simulink model "sampleModel7"  (R2021a)
settings: Solver=VariableStepAuto  StartTime=0.0  StopTime=10.0  RelTol=1e-3
undefined symbols (not defined in the file): DiscIntNeverNeededParam, magnitude, Newton, Raphson
libraries: simulink x210, pid_lib x47, simulink_need_slupdate x2
(part 7 of 8)

== system sampleModel7/cfblk364/cfblk6/cfblk16/cfblk5 ==
  cfblk1 : Inport
  cfblk15 : Inport  Port=2
  cfblk16 : Inport  Port=3
  cfblk10 : Sum  Inputs=|++
  cfblk11 : Sqrt  SaturateOnIntegerOverflow=on
  cfblk12 : Sin  TimeSource=Use external signal  SampleTime=0
  cfblk13 : Reshape
  cfblk14 : Sqrt  Operator=rSqrt  AlgorithmType=Newton-Raphson  SaturateOnIntegerOverflow=on
  cfblk17 : Delay
  cfblk3 : simulink/Discrete/Difference  ICPrevInput=0.0  OutMin=[]  OutMax=[]  OutDataTypeStr=Inherit: Inherit via back propagation  OutDataType=fixdt(1, 16)  OutScaling=2^-10  DoSatur=off
  cfblk4 : simulink/Discrete/Tapped Delay  vinit=0.0  samptime=-1  NumDelays=1  DelayOrder=Oldest  includeCurrent=off
  cfblk5 : DiscreteZeroPole  Poles=[0 0.5]  Gain=1  SampleTime=-1
  cfblk6 : Sqrt  Operator=rSqrt  AlgorithmType=Newton-Raphson  SaturateOnIntegerOverflow=on
  cfblk7 : Sum  Inputs=+-
  cfblk8 : DotProduct  InputSameDT=on  OutDataTypeStr=Inherit: Inherit via internal rule
  cfblk9 : MinMax  Function=max
  cfblk2 : Outport
  wires:
  cfblk13/1 -> cfblk10/1
  cfblk5/1 -> cfblk10/2
  cfblk11/1 -> cfblk7/1
  cfblk7/1 -> cfblk5/1
  cfblk16/1 -> cfblk6/1
  cfblk3/1 -> cfblk13/1, cfblk8/2
  cfblk12/1 -> cfblk2/1
  cfblk6/1 -> cfblk3/1
  cfblk9/1 -> cfblk12/1
  cfblk14/1 -> cfblk9/1
  cfblk15/1 -> cfblk14/1
  cfblk4/1 -> cfblk8/1
  cfblk1/1 -> cfblk4/1
  cfblk8/1 -> cfblk11/1
  cfblk10/1 -> cfblk17/1
  cfblk17/1 -> cfblk7/2

== system sampleModel7/cfblk364/cfblk6/cfblk16/cfblk6 ==
  cfblk1 : Inport
  cfblk7 : Inport  Port=2
  cfblk10 : Delay
  cfblk11 : Delay
  cfblk12 : Delay
  cfblk3 : DiscreteFir
  cfblk4 : Delay  DelayLengthSource=Input port
      settings: InputPortMap=u0,p1
  cfblk5 : Constant  Value=[426363474.539316]  SampleTime=1
  cfblk6 : If  IfExpression=u1 >= 0  SampleTime=1
  cfblk8 : Subsystem  TreatAsAtomicUnit=on
  cfblk9 : Subsystem  TreatAsAtomicUnit=on
  cfblk2 : Outport
  wires:
  cfblk1/1 -> cfblk9/2(cfblk12)
  cfblk7/1 -> cfblk9/3(cfblk13)
  cfblk5/1 -> cfblk6/1, cfblk8/2(cfblk14)
  cfblk9/1(cfblk2) -> cfblk4/2
  cfblk4/1 -> cfblk2/1, cfblk10/1
  cfblk9/2(cfblk14) -> cfblk8/1(cfblk1), cfblk8/3(cfblk15)
  cfblk8/2(cfblk17) -> cfblk3/1
  cfblk6/1 -> cfblk8/Action
  cfblk6/2 -> cfblk9/Action
  cfblk10/1 -> cfblk8/4(cfblk16)
  cfblk8/1(cfblk2) -> cfblk11/1
  cfblk11/1 -> cfblk9/1(cfblk1)
  cfblk3/1 -> cfblk12/1
  cfblk12/1 -> cfblk4/1

== system sampleModel7/cfblk382/cfblk17/cfblk13/cfblk6 ==
  cfblk1 : Inport
  cfblk7 : Inport  Port=2
  cfblk8 : Inport  Port=3
  cfblk3 : UnitDelay  SampleTime=-1  HasFrameUpgradeWarning=on
  cfblk4 : pid_lib/PID Controller  Controller=PID  Form=Parallel  TimeDomain=Discrete-time  UseExternalTs=off  SampleTime=-1  IntegratorMethod=Forward Euler  FilterMethod=Forward Euler  ControllerParametersSource=internal  P=1  I=1  D=0  UseFilter=on  N=100  TunerSelectOption=Transfer Function Based (PID Tuner App)  InitialConditionSource=internal  InitialConditionForIntegrator=0  InitialConditionForFilter=0  DifferentiatorICPrevScaledInput=0  ExternalReset=none  TrackingMode=off  Kt=1  LimitOutput=off  SatLimitsSource=internal  UpperSaturationLimit=inf  LowerSaturationLimit=-inf  LinearizeAsGain=off  AntiWindupMode=none  Kb=1  POutMin=[]  POutMax=[]  IOutMin=[]  IOutMax=[]  DOutMin=[]  DOutMax=[]  NOutMin=[]  NOutMax=[]  SumOutMin=[]  SumOutMax=[]  SaturationOutMin=[]  SaturationOutMax=[]  PParamMin=[]  PParamMax=[]  IParamMin=[]  IParamMax=[]  DParamMin=[]  DParamMax=[]  NParamMin=[]  NParamMax=[]  KbParamMin=[]  KbParamMax=[]  KtParamMin=[]  KtParamMax=[]  KbOutMin=[]  KbOutMax=[]  KtOutMin=[]  KtOutMax=[]  IntegratorOutMin=[]  IntegratorOutMax=[]  FilterOutMin=[]  FilterOutMax=[]  SumI1OutMin=[]  SumI1OutMax=[]  SumI2OutMin=[]  SumI2OutMax=[]  SumI3OutMin=[]  SumI3OutMax=[]  SumI4OutMin=[]  SumI4OutMax=[]  SumDOutMin=[]  SumDOutMax=[]  DifferentiatorOutMin=[]  DifferentiatorOutMax=[]  FilterDiffOutCoefMin=[]  FilterDiffOutCoefMax=[]  ReciprocalOutMin=[]  ReciprocalOutMax=[]  SumDenOutMin=[]  SumDenOutMax=[]  SumNumOutMin=[]  SumNumOutMax=[]  DivideOutMin=[]  DivideOutMax=[]  UdiffTsProdOutMin=[]  UdiffTsProdOutMax=[]  NTsProdOutMin=[]  NTsProdOutMax=[]  UintegralTsProdOutMin=[]  UintegralTsProdOutMax=[]  UngainTsProdOutMin=[]  UngainTsProdOutMax=[]  IntegratorContinuousStateAttributes=''  IntegratorStateMustResolveToSignalObject=off  IntegratorRTWStateStorageClass=Auto  FilterContinuousStateAttributes=''  FilterStateMustResolveToSignalObject=off  FilterRTWStateStorageClass=Auto  ParallelPVariant=InternalParameters  IdealPVariant=Disabled  IVariant=InternalParameters  DVariant=InternalParameters  IntegratorVariant=Discrete  SatVariant=Disabled  AWVariant=Passthrough  PCopyVariant=Disabled  TRVariant=Disabled  FdbkBlocksVariant=Forward  IdealPFdbkVariant=Disabled  SatFdbkVariant=Disabled  DerivativeFilterVariant=ForwardEulerFilter  NVariant=InternalParameters  NCopyVariant=Disabled  FilterICVariant=InternalICsFilter  IntegratorICVariant=InternalICs  ExternalResetVariant=Disabled  TRSumVariant=Passthrough  SumFdbkVariant=Disabled  SumVariant=Sum_PID  TsampFilterVariant=InternalTs  TsampNgainVariant=Passthrough  TsampIntegralVariant=Passthrough  ExternalSaturationOutDataTypeStr=Inherit: Same as second input
  cfblk5 : Sum  Inputs=+
  cfblk6 : Subsystem
  cfblk2 : Outport
  wires:
  cfblk1/1 -> cfblk6/1(cfblk1)
  cfblk4/1 -> cfblk5/1
  cfblk5/1 -> cfblk2/1
  cfblk7/1 -> cfblk6/2(cfblk9)
  cfblk6/1(cfblk2) -> cfblk3/1
  cfblk3/1 -> cfblk4/1

== system sampleModel7/cfblk384/cfblk14/cfblk8/cfblk11 ==
  cfblk1 : Inport
  cfblk8 : Inport  Port=2
  cfblk9 : Inport  Port=3
  cfblk10 : Inport  Port=4
  cfblk12 : Delay
  cfblk3 : Delay
  cfblk4 : DiscreteStateSpace  SampleTime=-1
  cfblk5 : DotProduct  InputSameDT=on  OutDataTypeStr=Inherit: Inherit via internal rule
  cfblk6 : Assignment  DiagnosticForDimensions=Warning  IndexOptions=Index vector (dialog)  Indices=1  OutputSizes=1
  cfblk7 : Constant  Value=[822552432.782879]  SampleTime=1
  cfblk2 : Outport
  cfblk11 : Outport  Port=2
  wires:
  cfblk7/1 -> cfblk2/1
  cfblk10/1 -> cfblk4/1
  cfblk1/1 -> cfblk11/1
  cfblk6/1 -> cfblk5/1
  cfblk4/1 -> cfblk3/1
  cfblk3/1 -> cfblk6/2
  cfblk9/1 -> cfblk5/2
  cfblk5/1 -> cfblk12/1
  cfblk12/1 -> cfblk6/1

== system sampleModel7/cfblk396/cfblk6/cfblk13/cfblk13 ==
  cfblk1 : Inport
  cfblk10 : Inport  Port=2
  cfblk11 : Inport  Port=3
  cfblk12 : Inport  Port=4
  cfblk3 : simulink/Discrete/Difference  ICPrevInput=0.0  OutMin=[]  OutMax=[]  OutDataTypeStr=Inherit: Inherit via back propagation  OutDataType=fixdt(1, 16)  OutScaling=2^-10  DoSatur=off
  cfblk4 : DiscreteFilter
  cfblk5 : Math  Operator=10^u  SaturateOnIntegerOverflow=on
  cfblk6 : Sum  Inputs=--
  cfblk7 : MinMax  Function=max  Inputs=3
  cfblk8 : Constant  Value=[446745629.042101]  SampleTime=1
  cfblk9 : Subsystem
  cfblk2 : Outport
  wires:
  cfblk4/1 -> cfblk9/1(cfblk1)
  cfblk10/1 -> cfblk6/1, cfblk7/3
  cfblk7/1 -> cfblk3/1
  cfblk8/1 -> cfblk7/1
  cfblk9/1(cfblk2) -> cfblk6/2
  cfblk12/1 -> cfblk5/1
  cfblk5/1 -> cfblk4/1
  cfblk3/1 -> cfblk9/2(cfblk8)
  cfblk6/1 -> cfblk2/1
  cfblk1/1 -> cfblk9/3(cfblk9)
  cfblk11/1 -> cfblk7/2

== system sampleModel7/cfblk399/cfblk15/cfblk6/cfblk8 ==
  cfblk1 : Inport
  cfblk10 : Inport  Port=2
  cfblk11 : Inport  Port=3
  cfblk12 : Inport  Port=4
  cfblk13 : Inport  Port=5
  cfblk14 : Inport  Port=6
  cfblk15 : DataTypeConversion
  cfblk3 : simulink/Discrete/Transfer Fcn First Order  PoleZ=0.95  ICPrevOutput=0.0  DoSatur=off
  cfblk4 : pid_lib/PID Controller  Controller=PID  Form=Parallel  TimeDomain=Discrete-time  UseExternalTs=off  SampleTime=-1  IntegratorMethod=Forward Euler  FilterMethod=Forward Euler  ControllerParametersSource=internal  P=1  I=1  D=0  UseFilter=on  N=100  TunerSelectOption=Transfer Function Based (PID Tuner App)  InitialConditionSource=internal  InitialConditionForIntegrator=0  InitialConditionForFilter=0  DifferentiatorICPrevScaledInput=0  ExternalReset=none  TrackingMode=off  Kt=1  LimitOutput=off  SatLimitsSource=internal  UpperSaturationLimit=inf  LowerSaturationLimit=-inf  LinearizeAsGain=off  AntiWindupMode=none  Kb=1  POutMin=[]  POutMax=[]  IOutMin=[]  IOutMax=[]  DOutMin=[]  DOutMax=[]  NOutMin=[]  NOutMax=[]  SumOutMin=[]  SumOutMax=[]  SaturationOutMin=[]  SaturationOutMax=[]  PParamMin=[]  PParamMax=[]  IParamMin=[]  IParamMax=[]  DParamMin=[]  DParamMax=[]  NParamMin=[]  NParamMax=[]  KbParamMin=[]  KbParamMax=[]  KtParamMin=[]  KtParamMax=[]  KbOutMin=[]  KbOutMax=[]  KtOutMin=[]  KtOutMax=[]  IntegratorOutMin=[]  IntegratorOutMax=[]  FilterOutMin=[]  FilterOutMax=[]  SumI1OutMin=[]  SumI1OutMax=[]  SumI2OutMin=[]  SumI2OutMax=[]  SumI3OutMin=[]  SumI3OutMax=[]  SumI4OutMin=[]  SumI4OutMax=[]  SumDOutMin=[]  SumDOutMax=[]  DifferentiatorOutMin=[]  DifferentiatorOutMax=[]  FilterDiffOutCoefMin=[]  FilterDiffOutCoefMax=[]  ReciprocalOutMin=[]  ReciprocalOutMax=[]  SumDenOutMin=[]  SumDenOutMax=[]  SumNumOutMin=[]  SumNumOutMax=[]  DivideOutMin=[]  DivideOutMax=[]  UdiffTsProdOutMin=[]  UdiffTsProdOutMax=[]  NTsProdOutMin=[]  NTsProdOutMax=[]  UintegralTsProdOutMin=[]  UintegralTsProdOutMax=[]  UngainTsProdOutMin=[]  UngainTsProdOutMax=[]  IntegratorContinuousStateAttributes=''  IntegratorStateMustResolveToSignalObject=off  IntegratorRTWStateStorageClass=Auto  FilterContinuousStateAttributes=''  FilterStateMustResolveToSignalObject=off  FilterRTWStateStorageClass=Auto  ParallelPVariant=InternalParameters  IdealPVariant=Disabled  IVariant=InternalParameters  DVariant=InternalParameters  IntegratorVariant=Discrete  SatVariant=Disabled  AWVariant=Passthrough  PCopyVariant=Disabled  TRVariant=Disabled  FdbkBlocksVariant=Forward  IdealPFdbkVariant=Disabled  SatFdbkVariant=Disabled  DerivativeFilterVariant=ForwardEulerFilter  NVariant=InternalParameters  NCopyVariant=Disabled  FilterICVariant=InternalICsFilter  IntegratorICVariant=InternalICs  ExternalResetVariant=Disabled  TRSumVariant=Passthrough  SumFdbkVariant=Disabled  SumVariant=Sum_PID  TsampFilterVariant=InternalTs  TsampNgainVariant=Passthrough  TsampIntegralVariant=Passthrough  ExternalSaturationOutDataTypeStr=Inherit: Same as second input
  cfblk5 : Product  Inputs=*
  cfblk6 : UnaryMinus
  cfblk7 : Constant  Value=[-757788657.864586]  SampleTime=1
  cfblk8 : Constant  Value=[-711690762.176715]  SampleTime=1
  cfblk9 : Constant  Value=[91822789.155668]  SampleTime=1
  cfblk2 : Outport
  wires:
  cfblk9/1 -> cfblk3/1
  cfblk7/1 -> cfblk6/1
  cfblk14/1 -> cfblk5/1
  cfblk3/1 -> cfblk2/1
  cfblk1/1 -> cfblk15/1
  cfblk15/1 -> cfblk4/1

== system sampleModel7/cfblk403/cfblk9/cfblk8/cfblk12 ==
  cfblk1 : Inport
  cfblk11 : Inport  Port=2
  cfblk12 : Inport  Port=3
  cfblk13 : Inport  Port=4
  cfblk14 : Inport  Port=5
  cfblk10 : Constant  Value=[-534013201.984926]  SampleTime=1
  cfblk3 : pid_lib/PID Controller  Controller=PID  Form=Parallel  TimeDomain=Discrete-time  UseExternalTs=off  SampleTime=-1  IntegratorMethod=Forward Euler  FilterMethod=Forward Euler  ControllerParametersSource=internal  P=1  I=1  D=0  UseFilter=on  N=100  TunerSelectOption=Transfer Function Based (PID Tuner App)  InitialConditionSource=internal  InitialConditionForIntegrator=0  InitialConditionForFilter=0  DifferentiatorICPrevScaledInput=0  ExternalReset=none  TrackingMode=off  Kt=1  LimitOutput=off  SatLimitsSource=internal  UpperSaturationLimit=inf  LowerSaturationLimit=-inf  LinearizeAsGain=off  AntiWindupMode=none  Kb=1  POutMin=[]  POutMax=[]  IOutMin=[]  IOutMax=[]  DOutMin=[]  DOutMax=[]  NOutMin=[]  NOutMax=[]  SumOutMin=[]  SumOutMax=[]  SaturationOutMin=[]  SaturationOutMax=[]  PParamMin=[]  PParamMax=[]  IParamMin=[]  IParamMax=[]  DParamMin=[]  DParamMax=[]  NParamMin=[]  NParamMax=[]  KbParamMin=[]  KbParamMax=[]  KtParamMin=[]  KtParamMax=[]  KbOutMin=[]  KbOutMax=[]  KtOutMin=[]  KtOutMax=[]  IntegratorOutMin=[]  IntegratorOutMax=[]  FilterOutMin=[]  FilterOutMax=[]  SumI1OutMin=[]  SumI1OutMax=[]  SumI2OutMin=[]  SumI2OutMax=[]  SumI3OutMin=[]  SumI3OutMax=[]  SumI4OutMin=[]  SumI4OutMax=[]  SumDOutMin=[]  SumDOutMax=[]  DifferentiatorOutMin=[]  DifferentiatorOutMax=[]  FilterDiffOutCoefMin=[]  FilterDiffOutCoefMax=[]  ReciprocalOutMin=[]  ReciprocalOutMax=[]  SumDenOutMin=[]  SumDenOutMax=[]  SumNumOutMin=[]  SumNumOutMax=[]  DivideOutMin=[]  DivideOutMax=[]  UdiffTsProdOutMin=[]  UdiffTsProdOutMax=[]  NTsProdOutMin=[]  NTsProdOutMax=[]  UintegralTsProdOutMin=[]  UintegralTsProdOutMax=[]  UngainTsProdOutMin=[]  UngainTsProdOutMax=[]  IntegratorContinuousStateAttributes=''  IntegratorStateMustResolveToSignalObject=off  IntegratorRTWStateStorageClass=Auto  FilterContinuousStateAttributes=''  FilterStateMustResolveToSignalObject=off  FilterRTWStateStorageClass=Auto  ParallelPVariant=InternalParameters  IdealPVariant=Disabled  IVariant=InternalParameters  DVariant=InternalParameters  IntegratorVariant=Discrete  SatVariant=Disabled  AWVariant=Passthrough  PCopyVariant=Disabled  TRVariant=Disabled  FdbkBlocksVariant=Forward  IdealPFdbkVariant=Disabled  SatFdbkVariant=Disabled  DerivativeFilterVariant=ForwardEulerFilter  NVariant=InternalParameters  NCopyVariant=Disabled  FilterICVariant=InternalICsFilter  IntegratorICVariant=InternalICs  ExternalResetVariant=Disabled  TRSumVariant=Passthrough  SumFdbkVariant=Disabled  SumVariant=Sum_PID  TsampFilterVariant=InternalTs  TsampNgainVariant=Passthrough  TsampIntegralVariant=Passthrough  ExternalSaturationOutDataTypeStr=Inherit: Same as second input
  cfblk4 : Bias  Bias=[542628662.857885]
  cfblk5 : Bias  Bias=[-760541575.504912]
  cfblk6 : Polyval  Coefs=[ +2.081618890e-019, -1.441693666e-014, +4.719686976e-010, -8.536869453e-006, +1.621573104e-001, -8.087801117e+001 ]
  cfblk7 : Sqrt  SaturateOnIntegerOverflow=on
  cfblk8 : UnaryMinus
  cfblk9 : MinMax  Function=max  Inputs=2
  cfblk2 : Outport
  wires:
  cfblk8/1 -> cfblk9/1
  cfblk10/1 -> cfblk8/1
  cfblk1/1 -> cfblk4/1
  cfblk12/1 -> cfblk2/1
  cfblk11/1 -> cfblk7/1
  cfblk13/1 -> cfblk6/1
  cfblk4/1 -> cfblk9/2
  cfblk9/1 -> cfblk5/1
  cfblk14/1 -> cfblk3/1

== system sampleModel7/cfblk349/cfblk10/cfblk10/cfblk10/cfblk13 ==
  cfblk1 : Inport
  cfblk9 : Inport  Port=2
  cfblk10 : Delay  SampleTime=1
  cfblk3 : Delay  ShowEnablePort=on  SampleTime=1
      settings: InputPortMap=u0,e6
  cfblk4 : Signum
  cfblk5 : Product
  cfblk6 : ComplexToMagnitudeAngle
  cfblk7 : Product  Inputs=**
  cfblk8 : Constant  Value=[-509073102.910421]  SampleTime=1
  cfblk2 : Outport
  wires:
  cfblk7/1 -> cfblk6/1
  cfblk6/1 -> cfblk5/1
  cfblk5/1 -> cfblk3/1
  cfblk8/1 -> cfblk3/2
  cfblk4/1 -> cfblk5/2
  cfblk9/1 -> cfblk4/1
  cfblk1/1 -> cfblk7/2
  cfblk3/1 -> cfblk2/1
  cfblk6/2 -> cfblk10/1
  cfblk10/1 -> cfblk7/1

== system sampleModel7/cfblk349/cfblk10/cfblk10/cfblk10/cfblk14 ==
  cfblk1 : Inport
  cfblk3 : Sin  TimeSource=Use external signal  SampleTime=0
  cfblk4 : Signum
  cfblk5 : UnaryMinus
  cfblk6 : Constant  Value=[-85370784.622687]  SampleTime=1
  cfblk7 : Constant  Value=[764398997.464723]  SampleTime=1
  cfblk2 : Outport
  wires:
  cfblk7/1 -> cfblk5/1
  cfblk1/1 -> cfblk3/1
  cfblk6/1 -> cfblk4/1
  cfblk4/1 -> cfblk2/1

== system sampleModel7/cfblk349/cfblk10/cfblk9/cfblk6/cfblk7 ==
  cfblk1 : Inport
  cfblk10 : Inport  Port=2
  cfblk11 : Inport  Port=3
  cfblk12 : Inport  Port=4
  cfblk3 : pid_lib/PID Controller (2DOF)  Controller=PID  Form=Parallel  TimeDomain=Discrete-time  UseExternalTs=off  SampleTime=1  IntegratorMethod=Forward Euler  FilterMethod=Forward Euler  ControllerParametersSource=internal  P=1  I=1  D=0  UseFilter=on  N=100  b=1  c=1  TunerSelectOption=Transfer Function Based (PID Tuner App)  InitialConditionSource=internal  InitialConditionForIntegrator=0  InitialConditionForFilter=0  DifferentiatorICPrevScaledInput=0  ExternalReset=none  TrackingMode=off  Kt=1  LimitOutput=off  SatLimitsSource=internal  UpperSaturationLimit=inf  LowerSaturationLimit=-inf  LinearizeAsGain=off  AntiWindupMode=none  Kb=1  POutMin=[]  POutMax=[]  IOutMin=[]  IOutMax=[]  DOutMin=[]  DOutMax=[]  NOutMin=[]  NOutMax=[]  bOutMin=[]  bOutMax=[]  cOutMin=[]  cOutMax=[]  SumOutMin=[]  SumOutMax=[]  SaturationOutMin=[]  SaturationOutMax=[]  PParamMin=[]  PParamMax=[]  IParamMin=[]  IParamMax=[]  DParamMin=[]  DParamMax=[]  NParamMin=[]  NParamMax=[]  bParamMin=[]  bParamMax=[]  cParamMin=[]  cParamMax=[]  KbParamMin=[]  KbParamMax=[]  KtParamMin=[]  KtParamMax=[]  KbOutMin=[]  KbOutMax=[]  KtOutMin=[]  KtOutMax=[]  IntegratorOutMin=[]  IntegratorOutMax=[]  FilterOutMin=[]  FilterOutMax=[]  SumI1OutMin=[]  SumI1OutMax=[]  SumI2OutMin=[]  SumI2OutMax=[]  SumI3OutMin=[]  SumI3OutMax=[]  SumI4OutMin=[]  SumI4OutMax=[]  SumDOutMin=[]  SumDOutMax=[]  Sum1OutMin=[]  Sum1OutMax=[]  Sum2OutMin=[]  Sum2OutMax=[]  Sum3OutMin=[]  Sum3OutMax=[]  DifferentiatorOutMin=[]  DifferentiatorOutMax=[]  FilterDiffOutCoefMin=[]  FilterDiffOutCoefMax=[]  ReciprocalOutMin=[]  ReciprocalOutMax=[]  SumDenOutMin=[]  SumDenOutMax=[]  SumNumOutMin=[]  SumNumOutMax=[]  DivideOutMin=[]  DivideOutMax=[]  UdiffTsProdOutMin=[]  UdiffTsProdOutMax=[]  NTsProdOutMin=[]  NTsProdOutMax=[]  UintegralTsProdOutMin=[]  UintegralTsProdOutMax=[]  UngainTsProdOutMin=[]  UngainTsProdOutMax=[]  IntegratorContinuousStateAttributes=''  IntegratorStateMustResolveToSignalObject=off  IntegratorRTWStateStorageClass=Auto  FilterContinuousStateAttributes=''  FilterStateMustResolveToSignalObject=off  FilterRTWStateStorageClass=Auto  ParallelPVariant=InternalParameters  IdealPVariant=Disabled  IVariant=InternalParameters  DVariant=InternalParameters  bVariant=InternalParameters  cVariant=InternalParameters  IntegratorVariant=Discrete  SatVariant=Disabled  AWVariant=Passthrough  PCopyVariant=Disabled  TRVariant=Disabled  FdbkBlocksVariant=Forward  IdealPFdbkVariant=Disabled  SatFdbkVariant=Disabled  DerivativeFilterVariant=ForwardEulerFilter  NVariant=InternalParameters  NCopyVariant=Disabled  FilterICVariant=InternalICsFilter  IntegratorICVariant=InternalICs  ExternalResetVariant=Disabled  TRSumVariant=Passthrough  SumFdbkVariant=Disabled  SumVariant=Sum_PID  TsampFilterVariant=InternalTs  TsampNgainVariant=Passthrough  TsampIntegralVariant=Passthrough  ExternalSaturationOutDataTypeStr=Inherit: Same as second input
      settings: SourceProductBaseCode=SL
  cfblk4 : DiscreteStateSpace
  cfblk5 : Delay  SampleTime=1
  cfblk6 : DiscreteFilter  SampleTime=1
  cfblk7 : simulink/Discrete/Transfer Fcn First Order  PoleZ=0.95  ICPrevOutput=0.0  DoSatur=off
  cfblk8 : Sin  TimeSource=Use external signal  SampleTime=0
  cfblk9 : simulink/Math Operations/MinMax Running Resettable  Function=min  vinit=0.0
  cfblk2 : Outport
  wires:
  cfblk12/1 -> cfblk7/1
  cfblk6/1 -> cfblk8/1
  cfblk1/1 -> cfblk4/1
  cfblk7/1 -> cfblk9/1
  cfblk5/1 -> cfblk6/1
  cfblk10/1 -> cfblk9/2
  cfblk9/1 -> cfblk3/1
  cfblk8/1 -> cfblk2/1
  cfblk11/1 -> cfblk3/2
  cfblk3/1 -> cfblk5/1

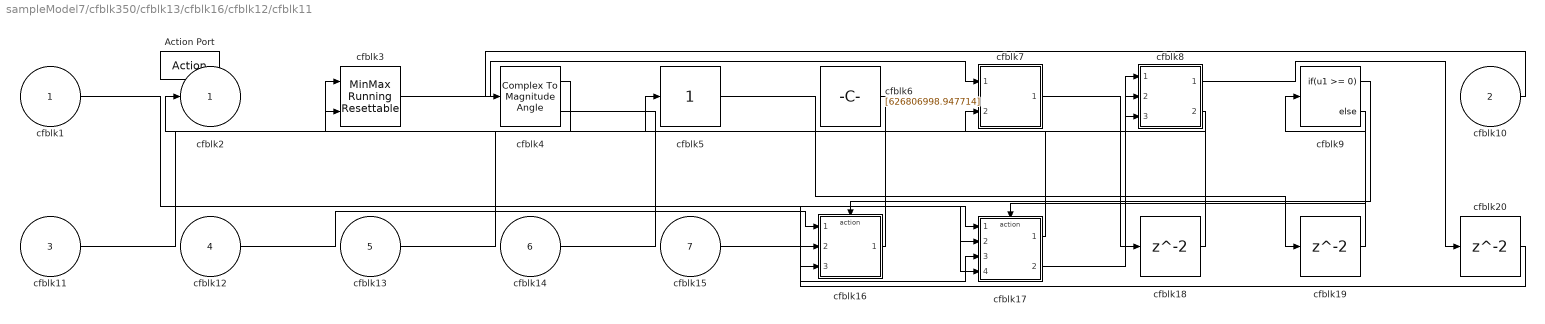
== system sampleModel7/cfblk350/cfblk13/cfblk16/cfblk12/cfblk11 ==
  cfblk1 : Inport
  cfblk10 : Inport  Port=2
  cfblk11 : Inport  Port=3
  cfblk12 : Inport  Port=4
  cfblk13 : Inport  Port=5
  cfblk14 : Inport  Port=6
  cfblk15 : Inport  Port=7
  Action Port : ActionPort  ActionPortLabel=if(u1 >= 0)
  cfblk16 : Subsystem  TreatAsAtomicUnit=on
  cfblk17 : Subsystem  TreatAsAtomicUnit=on
  cfblk18 : Delay
  cfblk19 : Delay
  cfblk20 : Delay
  cfblk3 : simulink/Math Operations/MinMax Running Resettable  Function=min  vinit=0.0
  cfblk4 : ComplexToMagnitudeAngle
  cfblk5 : simulink/Math Operations/Slider Gain  gain=1  low=0  high=2
  cfblk6 : Constant  Value=[626806998.947714]  SampleTime=1
  cfblk7 : Subsystem
  cfblk8 : Subsystem
  cfblk9 : If  IfExpression=u1 >= 0  SampleTime=1
  cfblk2 : Outport
  wires:
  cfblk17/1(cfblk2) -> cfblk5/1
  cfblk3/1 -> cfblk7/1(cfblk1)
  cfblk12/1 -> cfblk16/1(cfblk1)
  cfblk4/1 -> cfblk2/1
  cfblk10/1 -> cfblk4/1
  cfblk8/2(cfblk9) -> cfblk7/2(cfblk9)
  cfblk6/1 -> cfblk16/3(cfblk8)
  cfblk1/1 -> cfblk17/1(cfblk1)
  cfblk11/1 -> cfblk8/1(cfblk1)
  cfblk13/1 -> cfblk8/2(cfblk7)
  cfblk14/1 -> cfblk17/2(cfblk12)
  cfblk17/2(cfblk15) -> cfblk8/3(cfblk8)
  cfblk16/1(cfblk2) -> cfblk3/1
  cfblk15/1 -> cfblk17/3(cfblk13)
  cfblk4/2 -> cfblk17/4(cfblk14)
  cfblk9/1 -> cfblk16/Action
  cfblk9/2 -> cfblk17/Action
  cfblk7/1(cfblk2) -> cfblk18/1
  cfblk18/1 -> cfblk3/2
  cfblk5/1 -> cfblk19/1
  cfblk19/1 -> cfblk9/1
  cfblk8/1(cfblk2) -> cfblk20/1
  cfblk20/1 -> cfblk16/2(cfblk7)

== system sampleModel7/cfblk350/cfblk13/cfblk16/cfblk12/cfblk12 ==
  cfblk1 : Inport
  cfblk6 : Inport  Port=2
  cfblk7 : Inport  Port=3
  cfblk8 : Inport  Port=4
  cfblk9 : Inport  Port=5
  cfblk10 : Inport  Port=6
  Action Port : ActionPort  ActionPortLabel=else
  cfblk3 : UnaryMinus
  cfblk4 : Sum  Inputs=|++
  cfblk5 : Polyval  Coefs=[ +2.081618890e-019, -1.441693666e-014, +4.719686976e-010, -8.536869453e-006, +1.621573104e-001, -8.087801117e+001 ]
  cfblk2 : Outport
  wires:
  cfblk8/1 -> cfblk2/1
  cfblk3/1 -> cfblk4/1
  cfblk10/1 -> cfblk5/1
  cfblk9/1 -> cfblk4/2
  cfblk1/1 -> cfblk3/1

== system sampleModel7/cfblk350/cfblk13/cfblk17/cfblk6/cfblk18 ==
  cfblk1 : Inport
  cfblk11 : Inport  Port=2
  cfblk12 : Inport  Port=3
  cfblk13 : Inport  Port=4
  cfblk14 : Inport  Port=5
  cfblk15 : Inport  Port=6
  Action Port : ActionPort  ActionPortLabel=if(u1 >= 0)
  cfblk10 : Subsystem
  cfblk16 : Delay
  cfblk17 : Delay
  cfblk3 : DiscreteZeroPole  Poles=[0 0.5]  Gain=1  SampleTime=-1
  cfblk4 : Delay  DelayLengthSource=Input port
      settings: InputPortMap=u0,p1
  cfblk5 : Assignment  DiagnosticForDimensions=Warning  IndexOptions=Index vector (dialog)  Indices=1  OutputSizes=1
  cfblk6 : Sum  Inputs=+
  cfblk7 : Assignment  DiagnosticForDimensions=Warning  IndexOptions=Index vector (dialog)  Indices=1  OutputSizes=1
  cfblk8 : simulink/Math Operations/Slider Gain  gain=1  low=0  high=2
  cfblk9 : Constant  Value=[-20660821.855437]  SampleTime=1
  cfblk2 : Outport
  wires:
  cfblk8/1 -> cfblk2/1
  cfblk15/1 -> cfblk5/1
  cfblk4/1 -> cfblk7/2
  cfblk5/1 -> cfblk8/1
  cfblk13/1 -> cfblk5/2
  cfblk11/1 -> cfblk3/1
  cfblk3/1 -> cfblk10/1(cfblk1)
  cfblk1/1 -> cfblk10/2(cfblk8)
  cfblk7/1 -> cfblk6/1, cfblk16/1
  cfblk10/1(cfblk2) -> cfblk4/1
  cfblk14/1 -> cfblk10/4(cfblk10)
  cfblk9/1 -> cfblk4/2
  cfblk12/1 -> cfblk10/5(cfblk11)
  cfblk16/1 -> cfblk10/3(cfblk9)
  cfblk6/1 -> cfblk17/1
  cfblk17/1 -> cfblk7/1

== system sampleModel7/cfblk350/cfblk13/cfblk17/cfblk6/cfblk19 ==
  cfblk1 : Inport
  cfblk11 : Inport  Port=2
  cfblk12 : Inport  Port=3
  cfblk13 : Inport  Port=4
  cfblk14 : Inport  Port=5
  cfblk15 : Inport  Port=6
  Action Port : ActionPort  ActionPortLabel=else
  cfblk10 : Subsystem
  cfblk16 : Delay
  cfblk17 : Delay
  cfblk18 : Delay
  cfblk3 : DiscreteFilter
  cfblk4 : Delay  DelayLengthSource=Input port
      settings: InputPortMap=u0,p1
  cfblk5 : ComplexToRealImag
  cfblk6 : Signum
  cfblk7 : Bias  Bias=[41415960.158917]
  cfblk8 : Bias  Bias=[195329552.760084]
  cfblk9 : Subsystem
  cfblk2 : Outport
  wires:
  cfblk13/1 -> cfblk2/1
  cfblk15/1 -> cfblk4/1
  cfblk10/1(cfblk2) -> cfblk4/2
  cfblk1/1 -> cfblk6/1
  cfblk5/1 -> cfblk8/1
  cfblk11/1 -> cfblk10/1(cfblk1)
  cfblk5/2 -> cfblk3/1
  cfblk10/2(cfblk9) -> cfblk9/2(cfblk6)
  cfblk7/1 -> cfblk9/3(cfblk7)
  cfblk14/1 -> cfblk7/1
  cfblk9/1(cfblk2) -> cfblk5/1
  cfblk12/1 -> cfblk9/4(cfblk8)
  cfblk6/1 -> cfblk10/3(cfblk7)
  cfblk4/1 -> cfblk16/1
  cfblk16/1 -> cfblk10/2(cfblk6)
  cfblk8/1 -> cfblk17/1
  cfblk17/1 -> cfblk9/1(cfblk1)
  cfblk3/1 -> cfblk18/1
  cfblk18/1 -> cfblk10/4(cfblk8)

== system sampleModel7/cfblk353/cfblk8/cfblk11/cfblk7/cfblk6 ==
  cfblk1 : Inport
  cfblk11 : Inport  Port=2
  cfblk12 : Inport  Port=3
  cfblk13 : Inport  Port=4
  cfblk10 : If  IfExpression=u1 >= 0  SampleTime=1
  cfblk14 : Subsystem  TreatAsAtomicUnit=on
  cfblk15 : Subsystem  TreatAsAtomicUnit=on
  cfblk{5,16..18} (4 alike) : Delay  SampleTime=1
  cfblk3 : UnitDelay  HasFrameUpgradeWarning=on
  cfblk4 : simulink/Discrete/Difference  ICPrevInput=0.0  OutMin=[]  OutMax=[]  OutDataTypeStr=Inherit: Inherit via back propagation  OutDataType=fixdt(1, 16)  OutScaling=2^-10  DoSatur=off
  cfblk6 : Sum  Inputs=+
  cfblk7 : PermuteDimensions
  cfblk8 : MinMax  Inputs=3
  cfblk9 : DotProduct  InputSameDT=on  OutDataTypeStr=Inherit: Inherit via internal rule
  cfblk2 : Outport
  wires:
  cfblk14/1(cfblk2) -> cfblk6/1, cfblk18/1
  cfblk13/1 -> cfblk15/1(cfblk1)
  cfblk4/1 -> cfblk3/1, cfblk14/2(cfblk4)
  cfblk7/1 -> cfblk14/1(cfblk1)
  cfblk11/1 -> cfblk15/2(cfblk6), cfblk8/3, cfblk14/3(cfblk5), cfblk15/7(cfblk11)
  cfblk5/1 -> cfblk7/1
  cfblk3/1 -> cfblk15/3(cfblk7), cfblk2/1, cfblk14/5(cfblk7)
  cfblk12/1 -> cfblk5/1, cfblk15/4(cfblk8), cfblk15/5(cfblk9), cfblk14/4(cfblk6)
  cfblk1/1 -> cfblk9/1, cfblk15/6(cfblk10), cfblk15/8(cfblk12)
  cfblk9/1 -> cfblk8/2, cfblk15/9(cfblk13)
  cfblk8/1 -> cfblk4/1
  cfblk10/1 -> cfblk14/Action
  cfblk10/2 -> cfblk15/Action
  cfblk15/1(cfblk2) -> cfblk16/1
  cfblk16/1 -> cfblk9/2
  cfblk6/1 -> cfblk17/1
  cfblk17/1 -> cfblk8/1
  cfblk18/1 -> cfblk10/1

== system sampleModel7/cfblk354/cfblk18/cfblk11/cfblk8/cfblk14 ==
  cfblk1 : Inport
  cfblk3 : UnitDelay  SampleTime=-1  HasFrameUpgradeWarning=on
  cfblk4 : pid_lib/PID Controller  Controller=PID  Form=Parallel  TimeDomain=Discrete-time  UseExternalTs=off  SampleTime=-1  IntegratorMethod=Forward Euler  FilterMethod=Forward Euler  ControllerParametersSource=internal  P=1  I=1  D=0  UseFilter=on  N=100  TunerSelectOption=Transfer Function Based (PID Tuner App)  InitialConditionSource=internal  InitialConditionForIntegrator=0  InitialConditionForFilter=0  DifferentiatorICPrevScaledInput=0  ExternalReset=none  TrackingMode=off  Kt=1  LimitOutput=off  SatLimitsSource=internal  UpperSaturationLimit=inf  LowerSaturationLimit=-inf  LinearizeAsGain=off  AntiWindupMode=none  Kb=1  POutMin=[]  POutMax=[]  IOutMin=[]  IOutMax=[]  DOutMin=[]  DOutMax=[]  NOutMin=[]  NOutMax=[]  SumOutMin=[]  SumOutMax=[]  SaturationOutMin=[]  SaturationOutMax=[]  PParamMin=[]  PParamMax=[]  IParamMin=[]  IParamMax=[]  DParamMin=[]  DParamMax=[]  NParamMin=[]  NParamMax=[]  KbParamMin=[]  KbParamMax=[]  KtParamMin=[]  KtParamMax=[]  KbOutMin=[]  KbOutMax=[]  KtOutMin=[]  KtOutMax=[]  IntegratorOutMin=[]  IntegratorOutMax=[]  FilterOutMin=[]  FilterOutMax=[]  SumI1OutMin=[]  SumI1OutMax=[]  SumI2OutMin=[]  SumI2OutMax=[]  SumI3OutMin=[]  SumI3OutMax=[]  SumI4OutMin=[]  SumI4OutMax=[]  SumDOutMin=[]  SumDOutMax=[]  DifferentiatorOutMin=[]  DifferentiatorOutMax=[]  FilterDiffOutCoefMin=[]  FilterDiffOutCoefMax=[]  ReciprocalOutMin=[]  ReciprocalOutMax=[]  SumDenOutMin=[]  SumDenOutMax=[]  SumNumOutMin=[]  SumNumOutMax=[]  DivideOutMin=[]  DivideOutMax=[]  UdiffTsProdOutMin=[]  UdiffTsProdOutMax=[]  NTsProdOutMin=[]  NTsProdOutMax=[]  UintegralTsProdOutMin=[]  UintegralTsProdOutMax=[]  UngainTsProdOutMin=[]  UngainTsProdOutMax=[]  IntegratorContinuousStateAttributes=''  IntegratorStateMustResolveToSignalObject=off  IntegratorRTWStateStorageClass=Auto  FilterContinuousStateAttributes=''  FilterStateMustResolveToSignalObject=off  FilterRTWStateStorageClass=Auto  ParallelPVariant=InternalParameters  IdealPVariant=Disabled  IVariant=InternalParameters  DVariant=InternalParameters  IntegratorVariant=Discrete  SatVariant=Disabled  AWVariant=Passthrough  PCopyVariant=Disabled  TRVariant=Disabled  FdbkBlocksVariant=Forward  IdealPFdbkVariant=Disabled  SatFdbkVariant=Disabled  DerivativeFilterVariant=ForwardEulerFilter  NVariant=InternalParameters  NCopyVariant=Disabled  FilterICVariant=InternalICsFilter  IntegratorICVariant=InternalICs  ExternalResetVariant=Disabled  TRSumVariant=Passthrough  SumFdbkVariant=Disabled  SumVariant=Sum_PID  TsampFilterVariant=InternalTs  TsampNgainVariant=Passthrough  TsampIntegralVariant=Passthrough  ExternalSaturationOutDataTypeStr=Inherit: Same as second input
  cfblk5 : DiscreteStateSpace  SampleTime=-1
  cfblk6 : ComplexToRealImag
  cfblk7 : UnaryMinus
  cfblk8 : Delay
  cfblk2 : Outport
  wires:
  cfblk6/1 -> cfblk5/1
  cfblk7/1 -> cfblk6/1
  cfblk1/1 -> cfblk4/1
  cfblk3/1 -> cfblk7/1
  cfblk5/1 -> cfblk2/1
  cfblk6/2 -> cfblk8/1
  cfblk8/1 -> cfblk3/1

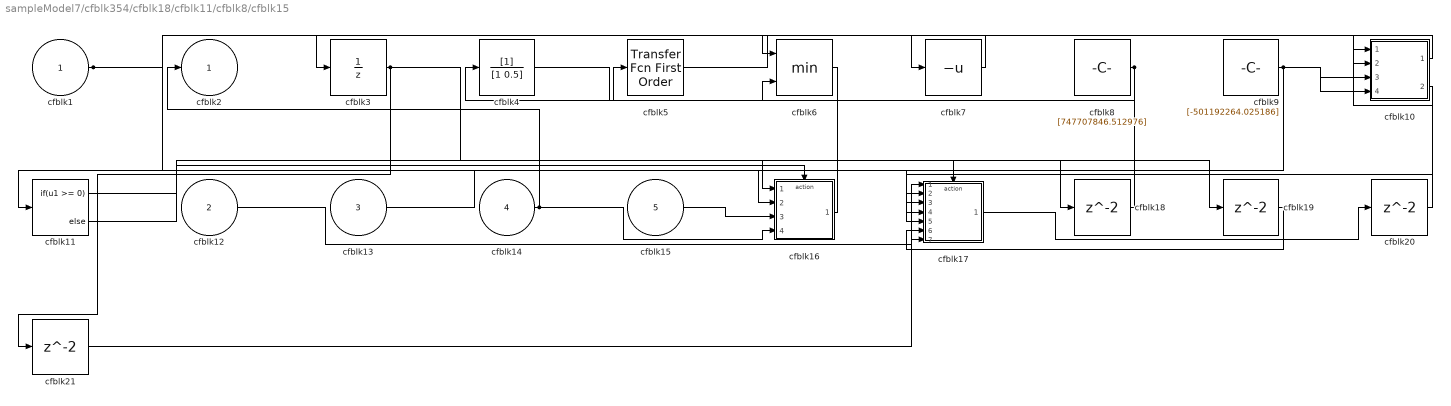
== system sampleModel7/cfblk354/cfblk18/cfblk11/cfblk8/cfblk15 ==
  cfblk1 : Inport
  cfblk12 : Inport  Port=2
  cfblk13 : Inport  Port=3
  cfblk14 : Inport  Port=4
  cfblk15 : Inport  Port=5
  cfblk10 : Subsystem
  cfblk11 : If  IfExpression=u1 >= 0  SampleTime=1
  cfblk16 : Subsystem  TreatAsAtomicUnit=on
  cfblk17 : Subsystem  TreatAsAtomicUnit=on
  cfblk{18..21} (4 alike) : Delay
  cfblk3 : UnitDelay  SampleTime=-1  HasFrameUpgradeWarning=on
  cfblk4 : DiscreteFilter
  cfblk5 : simulink/Discrete/Transfer Fcn First Order  PoleZ=0.95  ICPrevOutput=0.0  DoSatur=off
  cfblk6 : MinMax  Inputs=2
  cfblk7 : UnaryMinus
  cfblk8 : Constant  Value=[747707846.512976]  SampleTime=1
  cfblk9 : Constant  Value=[-501192264.025186]  SampleTime=1
  cfblk2 : Outport
  wires:
  cfblk7/1 -> cfblk3/1
  cfblk8/1 -> cfblk4/1, cfblk17/5(cfblk15)
  cfblk14/1 -> cfblk2/1, cfblk16/4(cfblk8)
  cfblk12/1 -> cfblk17/1(cfblk1)
  cfblk5/1 -> cfblk7/1
  cfblk3/1 -> cfblk18/1, cfblk19/1, cfblk21/1
  cfblk10/1(cfblk2) -> cfblk6/1
  cfblk6/1 -> cfblk11/1
  cfblk16/1(cfblk2) -> cfblk5/1
  cfblk4/1 -> cfblk6/2
  cfblk9/1 -> cfblk16/2(cfblk6), cfblk10/3(cfblk9), cfblk10/4(cfblk10)
  cfblk13/1 -> cfblk17/2(cfblk12)
  cfblk1/1 -> cfblk10/2(cfblk8), cfblk17/4(cfblk14)
  cfblk15/1 -> cfblk16/3(cfblk7)
  cfblk10/2(cfblk11) -> cfblk17/3(cfblk13)
  cfblk11/1 -> cfblk16/Action
  cfblk11/2 -> cfblk17/Action
  cfblk18/1 -> cfblk16/1(cfblk1)
  cfblk19/1 -> cfblk17/6(cfblk16)
  cfblk17/1(cfblk2) -> cfblk20/1
  cfblk20/1 -> cfblk10/1(cfblk1)
  cfblk21/1 -> cfblk17/7(cfblk17)

== system sampleModel7/cfblk364/cfblk6/cfblk16/cfblk4/cfblk15 ==
  cfblk1 : Inport
  cfblk10 : Inport  Port=2
  cfblk11 : Inport  Port=3
  Action Port : ActionPort  ActionPortLabel=if(u1 >= 0)
  cfblk12 : Delay
  cfblk3 : simulink/Discrete/Transfer Fcn First Order  PoleZ=0.95  ICPrevOutput=0.0  DoSatur=off
  cfblk4 : Sum  Inputs=-+
  cfblk5 : Product
  cfblk6 : Reshape
  cfblk7 : Reshape
  cfblk8 : Product  Inputs=*
  cfblk9 : Subsystem
  cfblk2 : Outport
  wires:
  cfblk6/1 -> cfblk2/1, cfblk9/3(cfblk9), cfblk9/4(cfblk10)
  cfblk11/1 -> cfblk5/1
  cfblk7/1 -> cfblk5/2
  cfblk1/1 -> cfblk4/2
  cfblk3/1 -> cfblk8/1
  cfblk10/1 -> cfblk3/1, cfblk9/2(cfblk8), cfblk9/5(cfblk11)
  cfblk4/1 -> cfblk7/1
  cfblk5/1 -> cfblk9/1(cfblk1)
  cfblk8/1 -> cfblk6/1
  cfblk9/1(cfblk2) -> cfblk12/1
  cfblk12/1 -> cfblk4/1

== system sampleModel7/cfblk364/cfblk6/cfblk16/cfblk4/cfblk16 ==
  cfblk1 : Inport
  cfblk8 : Inport  Port=2
  cfblk9 : Inport  Port=3
  Action Port : ActionPort  ActionPortLabel=else
  cfblk10 : Delay
  cfblk11 : Delay
  cfblk3 : Delay  ShowEnablePort=on
      settings: InputPortMap=u0,e6
  cfblk4 : pid_lib/PID Controller  Controller=PID  Form=Parallel  TimeDomain=Discrete-time  UseExternalTs=off  SampleTime=-1  IntegratorMethod=Forward Euler  FilterMethod=Forward Euler  ControllerParametersSource=internal  P=1  I=1  D=0  UseFilter=on  N=100  TunerSelectOption=Transfer Function Based (PID Tuner App)  InitialConditionSource=internal  InitialConditionForIntegrator=0  InitialConditionForFilter=0  DifferentiatorICPrevScaledInput=0  ExternalReset=none  TrackingMode=off  Kt=1  LimitOutput=off  SatLimitsSource=internal  UpperSaturationLimit=inf  LowerSaturationLimit=-inf  LinearizeAsGain=off  AntiWindupMode=none  Kb=1  POutMin=[]  POutMax=[]  IOutMin=[]  IOutMax=[]  DOutMin=[]  DOutMax=[]  NOutMin=[]  NOutMax=[]  SumOutMin=[]  SumOutMax=[]  SaturationOutMin=[]  SaturationOutMax=[]  PParamMin=[]  PParamMax=[]  IParamMin=[]  IParamMax=[]  DParamMin=[]  DParamMax=[]  NParamMin=[]  NParamMax=[]  KbParamMin=[]  KbParamMax=[]  KtParamMin=[]  KtParamMax=[]  KbOutMin=[]  KbOutMax=[]  KtOutMin=[]  KtOutMax=[]  IntegratorOutMin=[]  IntegratorOutMax=[]  FilterOutMin=[]  FilterOutMax=[]  SumI1OutMin=[]  SumI1OutMax=[]  SumI2OutMin=[]  SumI2OutMax=[]  SumI3OutMin=[]  SumI3OutMax=[]  SumI4OutMin=[]  SumI4OutMax=[]  SumDOutMin=[]  SumDOutMax=[]  DifferentiatorOutMin=[]  DifferentiatorOutMax=[]  FilterDiffOutCoefMin=[]  FilterDiffOutCoefMax=[]  ReciprocalOutMin=[]  ReciprocalOutMax=[]  SumDenOutMin=[]  SumDenOutMax=[]  SumNumOutMin=[]  SumNumOutMax=[]  DivideOutMin=[]  DivideOutMax=[]  UdiffTsProdOutMin=[]  UdiffTsProdOutMax=[]  NTsProdOutMin=[]  NTsProdOutMax=[]  UintegralTsProdOutMin=[]  UintegralTsProdOutMax=[]  UngainTsProdOutMin=[]  UngainTsProdOutMax=[]  IntegratorContinuousStateAttributes=''  IntegratorStateMustResolveToSignalObject=off  IntegratorRTWStateStorageClass=Auto  FilterContinuousStateAttributes=''  FilterStateMustResolveToSignalObject=off  FilterRTWStateStorageClass=Auto  ParallelPVariant=InternalParameters  IdealPVariant=Disabled  IVariant=InternalParameters  DVariant=InternalParameters  IntegratorVariant=Discrete  SatVariant=Disabled  AWVariant=Passthrough  PCopyVariant=Disabled  TRVariant=Disabled  FdbkBlocksVariant=Forward  IdealPFdbkVariant=Disabled  SatFdbkVariant=Disabled  DerivativeFilterVariant=ForwardEulerFilter  NVariant=InternalParameters  NCopyVariant=Disabled  FilterICVariant=InternalICsFilter  IntegratorICVariant=InternalICs  ExternalResetVariant=Disabled  TRSumVariant=Passthrough  SumFdbkVariant=Disabled  SumVariant=Sum_PID  TsampFilterVariant=InternalTs  TsampNgainVariant=Passthrough  TsampIntegralVariant=Passthrough  ExternalSaturationOutDataTypeStr=Inherit: Same as second input
  cfblk5 : simulink/Discrete/Tapped Delay  vinit=0.0  samptime=-1  NumDelays=1  DelayOrder=Oldest  includeCurrent=off
  cfblk6 : Sum  Inputs=+
  cfblk7 : Assignment  DiagnosticForDimensions=Warning  IndexOptions=Index vector (dialog)  Indices=1  OutputSizes=1
  cfblk2 : Outport
  wires:
  cfblk1/1 -> cfblk6/1
  cfblk8/1 -> cfblk2/1
  cfblk6/1 -> cfblk7/2
  cfblk7/1 -> cfblk5/1
  cfblk9/1 -> cfblk3/1
  cfblk3/1 -> cfblk4/1
  cfblk5/1 -> cfblk10/1
  cfblk10/1 -> cfblk7/1
  cfblk4/1 -> cfblk11/1
  cfblk11/1 -> cfblk3/2

== system sampleModel7/cfblk364/cfblk6/cfblk16/cfblk6/cfblk8 ==
  cfblk1 : Inport
  cfblk14 : Inport  Port=2
  cfblk15 : Inport  Port=3
  cfblk16 : Inport  Port=4
  Action Port : ActionPort  ActionPortLabel=if(u1 >= 0)
  cfblk10 : ComplexToRealImag
  cfblk11 : Constant  Value=[-112257015.331733]  SampleTime=1
  cfblk12 : Subsystem
  cfblk13 : Subsystem
  cfblk18 : Delay
  cfblk19 : Delay
  cfblk3 : UnitDelay  SampleTime=-1  HasFrameUpgradeWarning=on
  cfblk4 : Product  Inputs=**
  cfblk5 : ComplexToMagnitudeAngle
  cfblk6 : Signum
  cfblk7 : Abs
  cfblk8 : Signum
  cfblk9 : Sum  Inputs=|++
  cfblk2 : Outport
  cfblk17 : Outport  Port=2
  wires:
  cfblk5/1 -> cfblk10/1
  cfblk11/1 -> cfblk6/1
  cfblk5/2 -> cfblk8/1
  cfblk14/1 -> cfblk4/1, cfblk12/3(cfblk10), cfblk12/4(cfblk11)
  cfblk1/1 -> cfblk17/1
  cfblk3/1 -> cfblk4/2
  cfblk8/1 -> cfblk7/1
  cfblk4/1 -> cfblk2/1
  cfblk10/1 -> cfblk12/1(cfblk1)
  cfblk10/2 -> cfblk3/1
  cfblk6/1 -> cfblk12/2(cfblk9)
  cfblk16/1 -> cfblk13/1(cfblk1)
  cfblk12/1(cfblk2) -> cfblk9/2
  cfblk9/1 -> cfblk13/2(cfblk16)
  cfblk15/1 -> cfblk13/3(cfblk17)
  cfblk13/1(cfblk2) -> cfblk18/1
  cfblk18/1 -> cfblk9/1
  cfblk7/1 -> cfblk19/1
  cfblk19/1 -> cfblk5/1

== system sampleModel7/cfblk364/cfblk6/cfblk16/cfblk6/cfblk9 ==
  cfblk1 : Inport
  cfblk12 : Inport  Port=2
  cfblk13 : Inport  Port=3
  Action Port : ActionPort  ActionPortLabel=else
  cfblk10 : Constant  Value=[643582872.122553]  SampleTime=1
  cfblk11 : Constant  Value=[-283486214.818912]  SampleTime=1
  cfblk3 : DiscreteIntegrator  SampleTime=-1  ICPrevOutput=DiscIntNeverNeededParam  ICPrevScaledInput=DiscIntNeverNeededParam
  cfblk4 : simulink/Discrete/Transfer Fcn Real Zero  ZeroZ=0.75  ICPrevInput=0.0  DoSatur=off
      settings: SourceProductBaseCode=SL
  cfblk5 : Sqrt  Operator=rSqrt  AlgorithmType=Newton-Raphson  SaturateOnIntegerOverflow=on
  cfblk6 : simulink/Math Operations/MinMax Running Resettable  Function=min  vinit=0.0
  cfblk7 : simulink/Math Operations/Slider Gain  gain=1  low=0  high=2
  cfblk8 : UnaryMinus
  cfblk9 : Abs
  cfblk2 : Outport
  cfblk14 : Outport  Port=2
  wires:
  cfblk10/1 -> cfblk3/1
  cfblk1/1 -> cfblk2/1
  cfblk5/1 -> cfblk4/1
  cfblk12/1 -> cfblk9/1
  cfblk13/1 -> cfblk5/1
  cfblk3/1 -> cfblk6/1
  cfblk7/1 -> cfblk8/1
  cfblk6/1 -> cfblk14/1
  cfblk9/1 -> cfblk6/2
  cfblk11/1 -> cfblk7/1

== system sampleModel7/cfblk382/cfblk17/cfblk13/cfblk6/cfblk6 ==
  cfblk1 : Inport
  cfblk9 : Inport  Port=2
  cfblk{10..13} (4 alike) : Delay
  cfblk3 : DiscreteStateSpace  SampleTime=-1
  cfblk4 : Sqrt  SaturateOnIntegerOverflow=on
  cfblk5 : Sum  Inputs=+-
  cfblk6 : Sum  Inputs=-+
  cfblk7 : Constant  Value=[795709179.975378]  SampleTime=1
  cfblk8 : Subsystem
  cfblk2 : Outport
  wires:
  cfblk1/1 -> cfblk8/1(cfblk1), cfblk8/5(cfblk12)
  cfblk5/1 -> cfblk3/1
  cfblk6/1 -> cfblk4/1
  cfblk8/1(cfblk2) -> cfblk6/1
  cfblk3/1 -> cfblk12/1, cfblk13/1
  cfblk9/1 -> cfblk8/3(cfblk10), cfblk5/1, cfblk2/1
  cfblk4/1 -> cfblk5/2, cfblk10/1, cfblk11/1
  cfblk7/1 -> cfblk6/2, cfblk8/6(cfblk13)
  cfblk10/1 -> cfblk8/4(cfblk11)
  cfblk11/1 -> cfblk8/8(cfblk15)
  cfblk12/1 -> cfblk8/2(cfblk9)
  cfblk13/1 -> cfblk8/7(cfblk14)

== system sampleModel7/cfblk396/cfblk6/cfblk13/cfblk13/cfblk9 ==
  cfblk1 : Inport
  cfblk8 : Inport  Port=2
  cfblk9 : Inport  Port=3
  cfblk10 : Delay
  cfblk3 : Delay  DelayLengthSource=Input port
      settings: InputPortMap=u0,p1
  cfblk4 : DiscreteStateSpace  SampleTime=-1
  cfblk5 : UnitDelay  SampleTime=-1  HasFrameUpgradeWarning=on
  cfblk6 : Sqrt  Operator=rSqrt  AlgorithmType=Newton-Raphson  SaturateOnIntegerOverflow=on
  cfblk7 : Constant  Value=[-19757594.537292]  SampleTime=1
  cfblk2 : Outport
  wires:
  cfblk9/1 -> cfblk2/1
  cfblk5/1 -> cfblk4/1
  cfblk7/1 -> cfblk3/1
  cfblk3/1 -> cfblk5/1
  cfblk8/1 -> cfblk6/1
  cfblk4/1 -> cfblk10/1
  cfblk10/1 -> cfblk3/2

== system sampleModel7/cfblk350/cfblk13/cfblk16/cfblk12/cfblk11/cfblk16 ==
  cfblk1 : Inport
  cfblk7 : Inport  Port=2
  cfblk8 : Inport  Port=3
  Action Port : ActionPort  ActionPortLabel=if(u1 >= 0)
  cfblk3 : simulink/Discrete/Tapped Delay  vinit=0.0  samptime=-1  NumDelays=1  DelayOrder=Oldest  includeCurrent=off
  cfblk4 : DiscreteStateSpace  SampleTime=-1
  cfblk5 : DiscreteIntegrator  SampleTime=-1  ICPrevOutput=DiscIntNeverNeededParam  ICPrevScaledInput=DiscIntNeverNeededParam
  cfblk6 : Sum  Inputs=|++
  cfblk2 : Outport
  wires:
  cfblk4/1 -> cfblk6/1
  cfblk6/1 -> cfblk2/1
  cfblk5/1 -> cfblk4/1
  cfblk8/1 -> cfblk5/1
  cfblk1/1 -> cfblk6/2
  cfblk7/1 -> cfblk3/1

== system sampleModel7/cfblk350/cfblk13/cfblk16/cfblk12/cfblk11/cfblk17 ==
  cfblk1 : Inport
  cfblk12 : Inport  Port=2
  cfblk13 : Inport  Port=3
  cfblk14 : Inport  Port=4
  Action Port : ActionPort  ActionPortLabel=else
  cfblk10 : Product  Inputs=*
  cfblk11 : simulink/Math Operations/MinMax Running Resettable  Function=min  vinit=0.0
  cfblk3 : DiscreteFir
  cfblk4 : Delay  DelayLengthSource=Input port
      settings: InputPortMap=u0,p1
  cfblk5 : UnitDelay  SampleTime=-1  HasFrameUpgradeWarning=on
  cfblk6 : Rounding
  cfblk7 : Sqrt  Operator=rSqrt  AlgorithmType=Newton-Raphson  SaturateOnIntegerOverflow=on
  cfblk8 : PermuteDimensions
  cfblk9 : DotProduct  InputSameDT=on  OutDataTypeStr=Inherit: Inherit via internal rule
  cfblk2 : Outport
  cfblk15 : Outport  Port=2
  wires:
  cfblk10/1 -> cfblk7/1
  cfblk1/1 -> cfblk15/1
  cfblk9/1 -> cfblk5/1
  cfblk6/1 -> cfblk10/1
  cfblk5/1 -> cfblk4/1
  cfblk4/1 -> cfblk2/1
  cfblk7/1 -> cfblk4/2
  cfblk12/1 -> cfblk9/1
  cfblk8/1 -> cfblk11/1
  cfblk3/1 -> cfblk6/1
  cfblk13/1 -> cfblk11/2
  cfblk11/1 -> cfblk3/1
  cfblk14/1 -> cfblk9/2, cfblk8/1

== system sampleModel7/cfblk350/cfblk13/cfblk16/cfblk12/cfblk11/cfblk7 ==
  cfblk1 : Inport
  cfblk9 : Inport  Port=2
  cfblk10 : Delay
  cfblk3 : DiscreteFir
  cfblk4 : DiscreteFir
  cfblk5 : Delay  ShowEnablePort=on
      settings: InputPortMap=u0,e6
  cfblk6 : Polyval  Coefs=[ +2.081618890e-019, -1.441693666e-014, +4.719686976e-010, -8.536869453e-006, +1.621573104e-001, -8.087801117e+001 ]
  cfblk7 : Sin  TimeSource=Use external signal  SampleTime=0
  cfblk8 : UnaryMinus
  cfblk2 : Outport
  wires:
  cfblk8/1 -> cfblk2/1
  cfblk9/1 -> cfblk3/1
  cfblk1/1 -> cfblk6/1
  cfblk5/1 -> cfblk4/1
  cfblk7/1 -> cfblk5/1
  cfblk6/1 -> cfblk7/1
  cfblk3/1 -> cfblk8/1
  cfblk4/1 -> cfblk10/1
  cfblk10/1 -> cfblk5/2

== system sampleModel7/cfblk350/cfblk13/cfblk16/cfblk12/cfblk11/cfblk8 ==
  cfblk1 : Inport
  cfblk7 : Inport  Port=2
  cfblk8 : Inport  Port=3
  cfblk3 : Delay  ShowEnablePort=on
      settings: InputPortMap=u0,e6
  cfblk4 : Sqrt  SaturateOnIntegerOverflow=on
  cfblk5 : Sqrt  SaturateOnIntegerOverflow=on
  cfblk6 : Constant  Value=[-408479104.842576]  SampleTime=1
  cfblk2 : Outport
  cfblk9 : Outport  Port=2
  wires:
  cfblk6/1 -> cfblk9/1
  cfblk3/1 -> cfblk2/1
  cfblk7/1 -> cfblk3/1
  cfblk1/1 -> cfblk3/2
  cfblk4/1 -> cfblk5/1
  cfblk8/1 -> cfblk4/1

== system sampleModel7/cfblk350/cfblk13/cfblk17/cfblk6/cfblk18/cfblk10 ==
  cfblk1 : Inport
  cfblk8 : Inport  Port=2
  cfblk9 : Inport  Port=3
  cfblk10 : Inport  Port=4
  cfblk11 : Inport  Port=5
  cfblk12 : Delay
  cfblk3 : DiscreteStateSpace  SampleTime=-1
  cfblk4 : Product  Inputs=*
  cfblk5 : Gain  Gain=[313352730.255542]
  cfblk6 : ComplexToMagnitudeAngle
  cfblk7 : Constant  Value=[13055523.911014]  SampleTime=1
  cfblk2 : Outport
  wires:
  cfblk10/1 -> cfblk5/1
  cfblk4/1 -> cfblk6/1
  cfblk5/1 -> cfblk3/1
  cfblk1/1 -> cfblk2/1
  cfblk6/1 -> cfblk12/1
  cfblk12/1 -> cfblk4/1

== system sampleModel7/cfblk350/cfblk13/cfblk17/cfblk6/cfblk19/cfblk10 ==
  cfblk1 : Inport
  cfblk6 : Inport  Port=2
  cfblk7 : Inport  Port=3
  cfblk8 : Inport  Port=4
  cfblk3 : MinMax  Inputs=3
  cfblk4 : Sum  Inputs=+-
  cfblk5 : Assignment  DiagnosticForDimensions=Warning  IndexOptions=Index vector (dialog)  Indices=1  OutputSizes=1
  cfblk2 : Outport
  cfblk9 : Outport  Port=2
  wires:
  cfblk1/1 -> cfblk4/1
  cfblk4/1 -> cfblk2/1
  cfblk6/1 -> cfblk4/2
  cfblk7/1 -> cfblk5/1
  cfblk3/1 -> cfblk9/1
  cfblk8/1 -> cfblk5/2, cfblk3/2
  cfblk5/1 -> cfblk3/1, cfblk3/3

== system sampleModel7/cfblk350/cfblk13/cfblk17/cfblk6/cfblk19/cfblk9 ==
  cfblk1 : Inport
  cfblk6 : Inport  Port=2
  cfblk7 : Inport  Port=3
  cfblk8 : Inport  Port=4
  cfblk3 : DiscreteFilter
  cfblk4 : Sum  Inputs=-+
  cfblk5 : Constant  Value=[-108836114.249493]  SampleTime=1
  cfblk2 : Outport
  wires:
  cfblk1/1 -> cfblk4/1
  cfblk3/1 -> cfblk4/2
  cfblk7/1 -> cfblk2/1
  cfblk6/1 -> cfblk3/1

== system sampleModel7/cfblk353/cfblk8/cfblk11/cfblk7/cfblk6/cfblk14 ==
  cfblk1 : Inport
  cfblk4 : Inport  Port=2
  cfblk5 : Inport  Port=3
  cfblk6 : Inport  Port=4
  cfblk7 : Inport  Port=5
  Action Port : ActionPort  ActionPortLabel=if(u1 >= 0)
  cfblk3 : Constant  Value=[-606507586.060954]  SampleTime=1
  cfblk2 : Outport
  wires:
  cfblk1/1 -> cfblk2/1

== system sampleModel7/cfblk353/cfblk8/cfblk11/cfblk7/cfblk6/cfblk15 ==
  cfblk1 : Inport
  cfblk6 : Inport  Port=2
  cfblk7 : Inport  Port=3
  cfblk8 : Inport  Port=4
  cfblk9 : Inport  Port=5
  cfblk10 : Inport  Port=6
  cfblk11 : Inport  Port=7
  cfblk12 : Inport  Port=8
  cfblk13 : Inport  Port=9
  Action Port : ActionPort  ActionPortLabel=else
  cfblk3 : Delay  ShowEnablePort=on
      settings: InputPortMap=u0,e6
  cfblk4 : Constant  Value=[24433226.310679]  SampleTime=1
  cfblk5 : Constant  Value=[-997905176.213627]  SampleTime=1
  cfblk2 : Outport
  wires:
  cfblk12/1 -> cfblk2/1
  cfblk5/1 -> cfblk3/1
  cfblk7/1 -> cfblk3/2

== system sampleModel7/cfblk354/cfblk18/cfblk11/cfblk8/cfblk15/cfblk10 ==
  cfblk1 : Inport
  cfblk8 : Inport  Port=2
  cfblk9 : Inport  Port=3
  cfblk10 : Inport  Port=4
  cfblk3 : simulink/Discrete/Transfer Fcn Lead or Lag  PoleZ=0.95  ZeroZ=0.75  ICPrevOutput=0.0  ICPrevInput=0.0  DoSatur=off
      settings: SourceProductBaseCode=SL
  cfblk4 : Delay  ShowEnablePort=on
      settings: InputPortMap=u0,e6
  cfblk5 : Sqrt  SaturateOnIntegerOverflow=on
  cfblk6 : Reshape
  cfblk7 : Math  SaturateOnIntegerOverflow=on
  cfblk2 : Outport
  cfblk11 : Outport  Port=2
  wires:
  cfblk5/1 -> cfblk7/1
  cfblk7/1 -> cfblk2/1
  cfblk10/1 -> cfblk4/1
  cfblk4/1 -> cfblk11/1
  cfblk9/1 -> cfblk3/1
  cfblk8/1 -> cfblk5/1
  cfblk3/1 -> cfblk4/2
  cfblk1/1 -> cfblk6/1

== system sampleModel7/cfblk354/cfblk18/cfblk11/cfblk8/cfblk15/cfblk16 ==
  cfblk1 : Inport
  cfblk6 : Inport  Port=2
  cfblk7 : Inport  Port=3
  cfblk8 : Inport  Port=4
  Action Port : ActionPort  ActionPortLabel=if(u1 >= 0)
  cfblk3 : Sum  Inputs=|++
  cfblk4 : ComplexToMagnitudeAngle
  cfblk5 : Sqrt  SaturateOnIntegerOverflow=on
  cfblk2 : Outport
  wires:
  cfblk3/1 -> cfblk4/1
  cfblk7/1 -> cfblk5/1
  cfblk8/1 -> cfblk3/1
  cfblk1/1 -> cfblk3/2
  cfblk6/1 -> cfblk2/1

== system sampleModel7/cfblk354/cfblk18/cfblk11/cfblk8/cfblk15/cfblk17 ==
  cfblk1 : Inport
  cfblk12 : Inport  Port=2
  cfblk13 : Inport  Port=3
  cfblk14 : Inport  Port=4
  cfblk15 : Inport  Port=5
  cfblk16 : Inport  Port=6
  cfblk17 : Inport  Port=7
  Action Port : ActionPort  ActionPortLabel=else
  cfblk10 : Squeeze
  cfblk11 : Constant  Value=[-20112604.830398]  SampleTime=1
  cfblk3 : simulink/Discrete/Difference  ICPrevInput=0.0  OutMin=[]  OutMax=[]  OutDataTypeStr=Inherit: Inherit via back propagation  OutDataType=fixdt(1, 16)  OutScaling=2^-10  DoSatur=off
  cfblk4 : simulink/Discrete/Transfer Fcn Lead or Lag  PoleZ=0.95  ZeroZ=0.75  ICPrevOutput=0.0  ICPrevInput=0.0  DoSatur=off
      settings: SourceProductBaseCode=SL
  cfblk5 : Rounding
  cfblk6 : UnaryMinus
  cfblk7 : Product  Inputs=**
  cfblk8 : Sqrt  Operator=rSqrt  AlgorithmType=Newton-Raphson  SaturateOnIntegerOverflow=on
  cfblk9 : Sin  TimeSource=Use external signal  SampleTime=0
  cfblk2 : Outport
  wires:
  cfblk1/1 -> cfblk4/1
  cfblk14/1 -> cfblk2/1
  cfblk10/1 -> cfblk8/1
  cfblk6/1 -> cfblk9/1
  cfblk13/1 -> cfblk7/1
  cfblk17/1 -> cfblk3/1
  cfblk3/1 -> cfblk6/1
  cfblk8/1 -> cfblk7/2
  cfblk11/1 -> cfblk10/1
  cfblk15/1 -> cfblk5/1

== system sampleModel7/cfblk364/cfblk6/cfblk16/cfblk4/cfblk15/cfblk9 ==
  cfblk1 : Inport
  cfblk8 : Inport  Port=2
  cfblk9 : Inport  Port=3
  cfblk10 : Inport  Port=4
  cfblk11 : Inport  Port=5
  cfblk12 : Delay
  cfblk3 : pid_lib/PID Controller (2DOF)  Controller=PID  Form=Parallel  TimeDomain=Discrete-time  UseExternalTs=off  SampleTime=-1  IntegratorMethod=Forward Euler  FilterMethod=Forward Euler  ControllerParametersSource=internal  P=1  I=1  D=0  UseFilter=on  N=100  b=1  c=1  TunerSelectOption=Transfer Function Based (PID Tuner App)  InitialConditionSource=internal  InitialConditionForIntegrator=0  InitialConditionForFilter=0  DifferentiatorICPrevScaledInput=0  ExternalReset=none  TrackingMode=off  Kt=1  LimitOutput=off  SatLimitsSource=internal  UpperSaturationLimit=inf  LowerSaturationLimit=-inf  LinearizeAsGain=off  AntiWindupMode=none  Kb=1  POutMin=[]  POutMax=[]  IOutMin=[]  IOutMax=[]  DOutMin=[]  DOutMax=[]  NOutMin=[]  NOutMax=[]  bOutMin=[]  bOutMax=[]  cOutMin=[]  cOutMax=[]  SumOutMin=[]  SumOutMax=[]  SaturationOutMin=[]  SaturationOutMax=[]  PParamMin=[]  PParamMax=[]  IParamMin=[]  IParamMax=[]  DParamMin=[]  DParamMax=[]  NParamMin=[]  NParamMax=[]  bParamMin=[]  bParamMax=[]  cParamMin=[]  cParamMax=[]  KbParamMin=[]  KbParamMax=[]  KtParamMin=[]  KtParamMax=[]  KbOutMin=[]  KbOutMax=[]  KtOutMin=[]  KtOutMax=[]  IntegratorOutMin=[]  IntegratorOutMax=[]  FilterOutMin=[]  FilterOutMax=[]  SumI1OutMin=[]  SumI1OutMax=[]  SumI2OutMin=[]  SumI2OutMax=[]  SumI3OutMin=[]  SumI3OutMax=[]  SumI4OutMin=[]  SumI4OutMax=[]  SumDOutMin=[]  SumDOutMax=[]  Sum1OutMin=[]  Sum1OutMax=[]  Sum2OutMin=[]  Sum2OutMax=[]  Sum3OutMin=[]  Sum3OutMax=[]  DifferentiatorOutMin=[]  DifferentiatorOutMax=[]  FilterDiffOutCoefMin=[]  FilterDiffOutCoefMax=[]  ReciprocalOutMin=[]  ReciprocalOutMax=[]  SumDenOutMin=[]  SumDenOutMax=[]  SumNumOutMin=[]  SumNumOutMax=[]  DivideOutMin=[]  DivideOutMax=[]  UdiffTsProdOutMin=[]  UdiffTsProdOutMax=[]  NTsProdOutMin=[]  NTsProdOutMax=[]  UintegralTsProdOutMin=[]  UintegralTsProdOutMax=[]  UngainTsProdOutMin=[]  UngainTsProdOutMax=[]  IntegratorContinuousStateAttributes=''  IntegratorStateMustResolveToSignalObject=off  IntegratorRTWStateStorageClass=Auto  FilterContinuousStateAttributes=''  FilterStateMustResolveToSignalObject=off  FilterRTWStateStorageClass=Auto  ParallelPVariant=InternalParameters  IdealPVariant=Disabled  IVariant=InternalParameters  DVariant=InternalParameters  bVariant=InternalParameters  cVariant=InternalParameters  IntegratorVariant=Discrete  SatVariant=Disabled  AWVariant=Passthrough  PCopyVariant=Disabled  TRVariant=Disabled  FdbkBlocksVariant=Forward  IdealPFdbkVariant=Disabled  SatFdbkVariant=Disabled  DerivativeFilterVariant=ForwardEulerFilter  NVariant=InternalParameters  NCopyVariant=Disabled  FilterICVariant=InternalICsFilter  IntegratorICVariant=InternalICs  ExternalResetVariant=Disabled  TRSumVariant=Passthrough  SumFdbkVariant=Disabled  SumVariant=Sum_PID  TsampFilterVariant=InternalTs  TsampNgainVariant=Passthrough  TsampIntegralVariant=Passthrough  ExternalSaturationOutDataTypeStr=Inherit: Same as second input
      settings: SourceProductBaseCode=SL
  cfblk4 : Rounding
  cfblk5 : Math  Operator=square  SaturateOnIntegerOverflow=on
  cfblk6 : Bias  Bias=[422634965.438158]
  cfblk7 : Product
  cfblk2 : Outport
  wires:
  cfblk6/1 -> cfblk7/1
  cfblk1/1 -> cfblk2/1
  cfblk9/1 -> cfblk7/2
  cfblk10/1 -> cfblk5/1
  cfblk5/1 -> cfblk4/1
  cfblk11/1 -> cfblk3/2
  cfblk3/1 -> cfblk6/1
  cfblk7/1 -> cfblk12/1
  cfblk12/1 -> cfblk3/1
